simulink model "tfschema5"  (Simulink 7.0)
settings: Solver=ode45  StartTime=Startt  StopTime=Stoptt  RelTol=1e-3
undefined symbols (not defined in the file or in its folder): DenC, DenG, Fve, FvPs, FvPu, Ive, IvPs, IvPu, NumC, NumG, Stepte, SteptPs, SteptPu
settings Model: Creator=pmelchio  LastModifiedBy=pmelchio

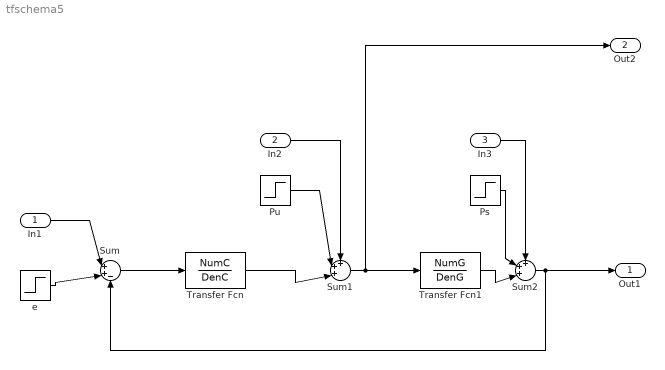
== system tfschema5 ==
  In1 : Inport  OutDataType=sfix(16)  OutScaling=2^0
  In2 : Inport  Port=2  OutDataType=sfix(16)  OutScaling=2^0
  In3 : Inport  Port=3  OutDataType=sfix(16)  OutScaling=2^0
  Ps : Step  Time=SteptPs  Before=IvPs  After=FvPs  SampleTime=0
  Pu : Step  Time=SteptPu  Before=IvPu  After=FvPu  SampleTime=0
  Sum : Sum  Inputs=|++-  OutDataType=sfix(16)  OutScaling=2^0
  Sum1 : Sum  Inputs=+++|  OutDataType=sfix(16)  OutScaling=2^0
  Sum2 : Sum  Inputs=+++|  OutDataType=sfix(16)  OutScaling=2^0
  Transfer Fcn : TransferFcn  Numerator=NumC  Denominator=DenC
  Transfer Fcn1 : TransferFcn  Numerator=NumG  Denominator=DenG
  e : Step  Time=Stepte  Before=Ive  After=Fve  SampleTime=0
  Out1 : Outport  OutDataType=sfix(16)  OutScaling=2^0
  Out2 : Outport  Port=2  OutDataType=sfix(16)  OutScaling=2^0
  wires:
  Sum1/1 -> Transfer Fcn1/1, Out2/1
  Sum/1 -> Transfer Fcn/1
  Sum2/1 -> Sum/3, Out1/1
  In1/1 -> Sum/1
  Transfer Fcn/1 -> Sum1/3
  Pu/1 -> Sum1/2
  In2/1 -> Sum1/1
  Ps/1 -> Sum2/2
  Transfer Fcn1/1 -> Sum2/3
  In3/1 -> Sum2/1
  e/1 -> Sum/2
